simulink model "Simulink_Modell"  (R2017b)
settings: Solver=VariableStepAuto  StartTime=0.0  StopTime=10.0  RelTol=1e-3
values from neighbouring files (symbols this model uses):
  A = double(vpa(A))    [Skript_Vorbereitung.m]
  b = double(vpa(b))    [Skript_Vorbereitung.m]
  C = [1 0 0 0; 0 0 1 0]    [Skript_Vorbereitung.m]
  k = acker(A,b,p)    [Skript_Vorbereitung.m]
undefined symbols (not defined in the file or in its folder): L
settings Model: Creator=Lucas  LastModifiedBy=Lucas

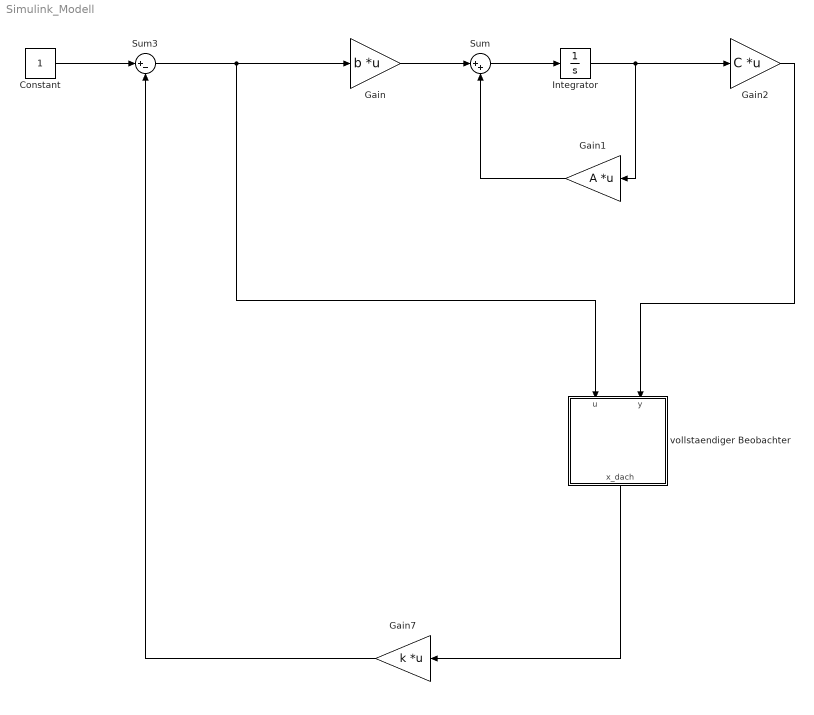
== system Simulink_Modell ==
  Constant : Constant
  Gain : Gain  Gain=b  Multiplication=Matrix(K*u)
  Gain1 : Gain  Gain=A  Multiplication=Matrix(K*u)
  Gain2 : Gain  Gain=C  Multiplication=Matrix(K*u)
  Gain7 : Gain  Gain=k  Multiplication=Matrix(K*u)
  Integrator : Integrator
  Sum : Sum  Inputs=|++
  Sum3 : Sum  Inputs=|+-
  vollstaendiger Beobachter : Subsystem
  wires:
  Gain/1 -> Sum/1
  Sum/1 -> Integrator/1
  Integrator/1 -> Gain2/1, Gain1/1
  Gain1/1 -> Sum/2
  Constant/1 -> Sum3/1
  Sum3/1 -> vollstaendiger Beobachter/1(u), Gain/1
  Gain7/1 -> Sum3/2
  Gain2/1 -> vollstaendiger Beobachter/2(y)
  vollstaendiger Beobachter/1(x_dach) -> Gain7/1

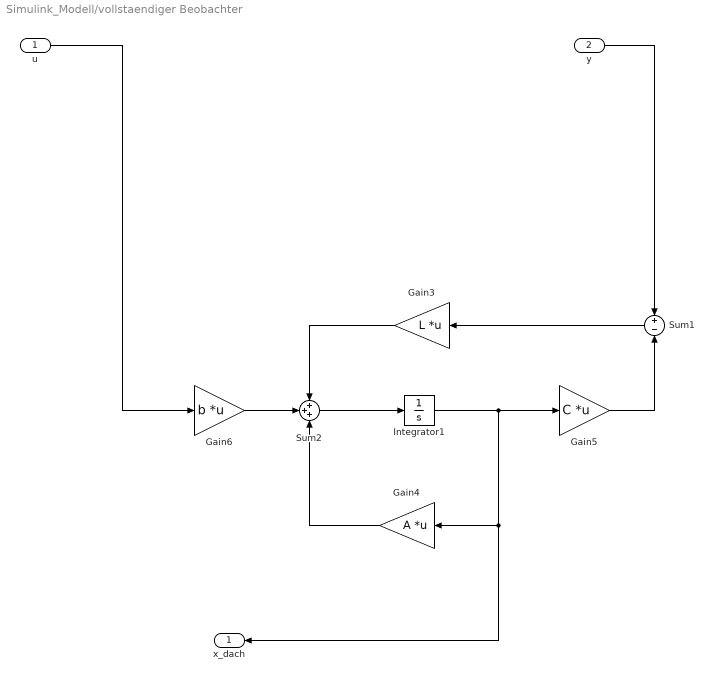
== system Simulink_Modell/vollstaendiger Beobachter ==
  u : Inport
  y : Inport  Port=2
  Gain3 : Gain  Gain=L  Multiplication=Matrix(K*u)
  Gain4 : Gain  Gain=A  Multiplication=Matrix(K*u)
  Gain5 : Gain  Gain=C  Multiplication=Matrix(K*u)
  Gain6 : Gain  Gain=b  Multiplication=Matrix(K*u)
  Integrator1 : Integrator
  Sum1 : Sum  Inputs=+-
  Sum2 : Sum  Inputs=+++
  x_dach : Outport
  wires:
  Gain3/1 -> Sum2/1
  Gain5/1 -> Sum1/2
  Sum1/1 -> Gain3/1
  u/1 -> Gain6/1
  y/1 -> Sum1/1
  Gain6/1 -> Sum2/2
  Integrator1/1 -> x_dach/1, Gain4/1, Gain5/1
  Sum2/1 -> Integrator1/1
  Gain4/1 -> Sum2/3
